simulink model "ControlClasico"  (Simulink 7.9)
settings: Solver=ode45  StartTime=0.0  StopTime=10.0  RelTol=1e-3
undefined symbols (not defined in the file or in its folder): k
libraries: simulink x1
settings Model: Creator=root  LastModifiedBy=root
settings ConfigComp: Description=Design Verifier Custom Configuration Component  DVMaxTestCaseSteps=500  DVTestSuiteOptimization=CombinedObjectives (Nonlinear Extended)

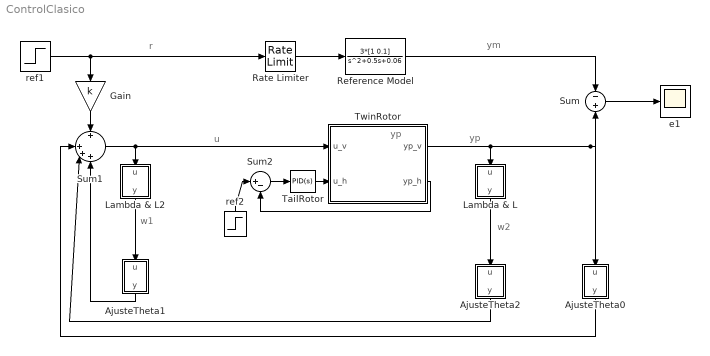
== system ControlClasico ==
  note: u
  note: r
  note: yp
  note: ym
  note: w2
  note: w1
  note: yp
  AjusteTheta0 : MATLAB Function  TreatAsAtomicUnit=on
  AjusteTheta1 : MATLAB Function  TreatAsAtomicUnit=on
  AjusteTheta2 : MATLAB Function  TreatAsAtomicUnit=on
  Gain : Gain  Gain=k
  Lambda & L : MATLAB Function  TreatAsAtomicUnit=on
  Lambda & L2 : MATLAB Function  TreatAsAtomicUnit=on
  Rate Limiter : RateLimiter  SampleTimeMode=inherited
  Reference Model : TransferFcn  Numerator=3*[1 0.1]  Denominator=[1 0.5 0.06]
  Sum : Sum  Inputs=-|+
  Sum1 : Sum  Inputs=+|+++
  Sum2 : Sum  Inputs=|+-
  TailRotor : simulink/Continuous/PID Controller  Controller=PID  TimeDomain=Continuous-time  SampleTime=1  IntegratorMethod=Forward Euler  FilterMethod=Forward Euler  Form=Parallel  P=8.4e-6  I=4.3e-6  D=0  N=100  InitialConditionSource=internal  InitialConditionForIntegrator=0  InitialConditionForFilter=0  ExternalReset=none  LimitOutput=off  UpperSaturationLimit=inf  LowerSaturationLimit=-inf  LinearizeAsGain=off  AntiWindupMode=none  Kb=1  TrackingMode=off  Kt=1  PParamMin=[]  PParamMax=[]  IParamMin=[]  IParamMax=[]  DParamMin=[]  DParamMax=[]  NParamMin=[]  NParamMax=[]  KbParamMin=[]  KbParamMax=[]  KtParamMin=[]  KtParamMax=[]  POutMin=[]  POutMax=[]  IOutMin=[]  IOutMax=[]  DOutMin=[]  DOutMax=[]  NOutMin=[]  NOutMax=[]  KbOutMin=[]  KbOutMax=[]  KtOutMin=[]  KtOutMax=[]  IntegratorOutMin=[]  IntegratorOutMax=[]  FilterOutMin=[]  FilterOutMax=[]  SumOutMin=[]  SumOutMax=[]  SumI1OutMin=[]  SumI1OutMax=[]  SumI2OutMin=[]  SumI2OutMax=[]  SumI3OutMin=[]  SumI3OutMax=[]  SumDOutMin=[]  SumDOutMax=[]  SaturationOutMin=[]  SaturationOutMax=[]  IntegratorContinuousStateAttributes=''  IntegratorStateMustResolveToSignalObject=off  IntegratorRTWStateStorageClass=Auto  FilterContinuousStateAttributes=''  FilterStateMustResolveToSignalObject=off  FilterRTWStateStorageClass=Auto
  TwinRotor : MATLAB Function  Description=imread('/home/hernan/Documentos/semestre10/labControl/repo/LaboratorioControlAvanzado/experiencia3/Twin-rotor-system.jpg')  LoadFcn=imread('/home/hernan/Documentos/semestre10/labControl/repo/LaboratorioControlAvanzado/experiencia3/Twin-rotor-system.jpg')  ClipboardFcn=imread('/home/hernan/Documentos/semestre10/labControl/repo/LaboratorioControlAvanzado/experiencia3/Twin-rotor-system.jpg')  TreatAsAtomicUnit=on
  e1 : Scope
      settings: SaveName=err1
  ref1 : Step  Time=0  After=4.7/1.88  SampleTime=0
  ref2 : Step  Time=0  After=4.7/1.88  SampleTime=0
  wires:
  Reference Model/1 -> Sum/1
  TwinRotor/1(yp_v) -> Sum/2, AjusteTheta0/1(u), Lambda & L/1(u)
  Sum1/1 -> TwinRotor/1(u_v), Lambda & L2/1(u)
  ref1/1 -> Rate Limiter/1, Gain/1
  Gain/1 -> Sum1/1
  Sum/1 -> e1/1
  Lambda & L2/1(y) -> AjusteTheta1/1(u)
  Lambda & L/1(y) -> AjusteTheta2/1(u)
  AjusteTheta1/1(y) -> Sum1/4
  AjusteTheta2/1(y) -> Sum1/3
  AjusteTheta0/1(y) -> Sum1/2
  Rate Limiter/1 -> Reference Model/1
  TailRotor/1 -> TwinRotor/2(u_h)
  Sum2/1 -> TailRotor/1
  ref2/1 -> Sum2/1
  TwinRotor/2(yp_h) -> Sum2/2

== matlab function AjusteTheta2 ==
  data: u input double; y output double
function y = fcn(u)
%#codegen

y = u;

== matlab function Lambda & L ==
  data: u input double; y output double
function y = fcn(u)
%#codegen

y = u;

== matlab function AjusteTheta0 ==
  data: u input double; y output double
function y = fcn(u)
%#codegen

y = u;

== matlab function TwinRotor ==
  data: u_v input double; yp_v output double; u_h input double; yp_h output double
function [yp_v, yp_h] = TwinRotor(u_v, u_h)
%TwinRotor Model
    yp_v = u_v;
    yp_h = u_h;
end

== matlab function AjusteTheta1 ==
  data: u input double; y output double
function y = fcn(u)
%#codegen

y = u;

== matlab function Lambda & L2 ==
  data: u input double; y output double
function y = fcn(u)
%#codegen

y = u;
